simulink model "sampleModel1747_1_sub"  (R2023a)
settings: Solver=VariableStepAuto  StartTime=0.0  StopTime=10.0  RelTol=1e-3
libraries: hdlsllib x5, simulink x3
settings Model: Creator=user1  LastModifiedBy=user1

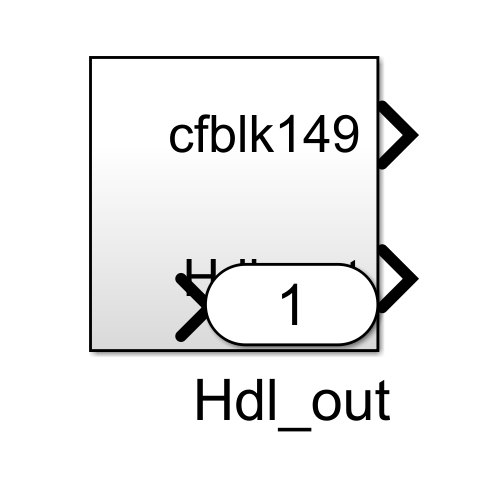
[thumbnail: Simulink's stored preview of the top-level diagram]
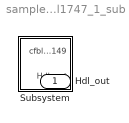
== system sampleModel1747_1_sub ==
  Subsystem : Subsystem
  Hdl_out : Outport  OutDataTypeStr=uint8

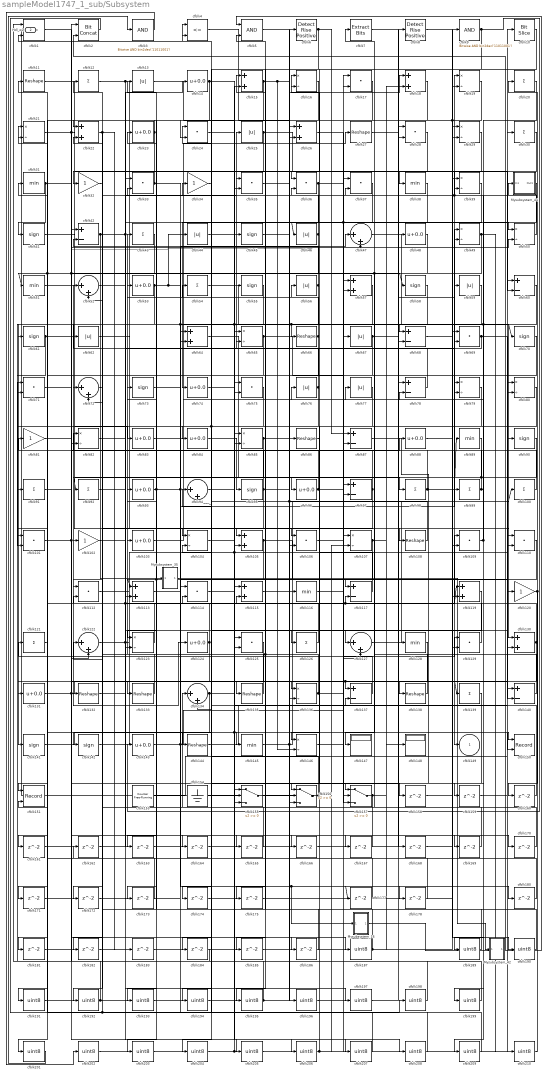
== system sampleModel1747_1_sub/Subsystem ==
  Mysubsystem_16 : Subsystem  TreatAsAtomicUnit=on  RTWFcnName=Mysubsystem_16
      settings: RTWFcnNameOpts=User specified  RTWFileNameOpts=Use function name
  Mysubsystem_35 : Subsystem  TreatAsAtomicUnit=on  RTWFcnName=Mysubsystem_35
      settings: RTWFcnNameOpts=User specified  RTWFileNameOpts=Use function name
  Mysubsystem_42 : Subsystem  TreatAsAtomicUnit=on  RTWFcnName=Mysubsystem_42
      settings: RTWFcnNameOpts=User specified  RTWFileNameOpts=Use function name
  Mysubsystem_44 : Subsystem  TreatAsAtomicUnit=on  RTWFcnName=Mysubsystem_44
      settings: RTWFcnNameOpts=User specified  RTWFileNameOpts=Use function name
  cfblk1 : RelationalOperator  Operator=<=  OutDataTypeStr=boolean  InputSameDT=off
  cfblk10 : hdlsllib/Logic and Bit Operations/Bit Slice  lidx=7  ridx=0
  cfblk{12,20,30,43,54,91..92,98..100,121,126,139} (13 alike) : Sum  Inputs=+  OutDataTypeStr=uint8
  cfblk{17,24,28,33,35..37,69,71,75,101,106,109..110,112,114,125,129} (18 alike) : DotProduct  OutDataTypeStr=uint8
  cfblk{32,34,81,102,120} (5 alike) : Gain  OutDataTypeStr=uint8
  cfblk{14,23,48,53,74,83..84,88,93,96,103,124,131,143} (14 alike) : Bias  Bias=0.0  SaturateOnIntegerOverflow=off
  cfblk{16,19,21,29,39,49..50,65,79..80,82,85,104,107,123,136,146} (17 alike) : Product  Inputs=*/  OutDataTypeStr=uint8  RndMeth=Zero  SaturateOnIntegerOverflow=on
  cfblk{15,18,22,26,57,64,105,113,115,119,130} (11 alike) : Sum  OutDataTypeStr=uint8
  cfblk{11,27,66,86,108,132..133,135,138,144} (10 alike) : Reshape
  cfblk{31,38,51,89,116,128,145} (7 alike) : MinMax  OutDataTypeStr=uint8
  cfblk{42,60,68,78,87,97,117,137,140} (9 alike) : Sum  Inputs=+-  OutDataTypeStr=uint8
  cfblk{47,52,72,94,122,127,134} (7 alike) : Sum  Inputs=|++  OutDataTypeStr=uint8
  cfblk{13,25,44,46,56,59,62,67,76..77} (10 alike) : Abs  OutDataTypeStr=uint8  SaturateOnIntegerOverflow=off
  cfblk{41,45,55,58,61,70,73,90,95,141..142} (11 alike) : Signum
  cfblk147 : Display
  cfblk148 : Display
  cfblk150 : Record  FileSettingsInternal="{\"entries\":[{\"content\":{\"excelSettings\":{\"content\":{},\"type\":\"Streamout.ExcelSettings\"}},\"type\":\"Streamout.FileSettingStorage\",\"uuid\":\"\"}],\"packageUris\":[\"http:\\/\\/schema.mathworks.com\\/mf0\\/streamout_blocks\\/R2020a\"],\"version\":\"1.0\"}"  Layout=[1 1]  SignalsInternal="{\"entries\":[{\"content\":{\"signals\":[{\"content\":{\"blockPath\":[],\"dimensions\":[1],\"domain\":\"\",\"lineColor\":\"#a2142f\",\"plots\":[1],\"port\":1,\"signalID\":39164,\"signalName\":\"cfblk36\"},\"type\":\"RecordBlkView.Signal\",\"uuid\":\"\"},{\"content\":{\"blockPath\":[],\"dimensions\":[1],\"domain\":\"\",\"lineColor\":\"#139fff\",\"plots\":[1],\"port\":2,\"signalID\":39167,\"signalName\":\"cfblk74\"},\"type\":\"RecordBlkView.Signal\",\"uuid\":\"\"}]},\"type\":\"RecordBlkView.InputSignals\",\"uuid\":\"\"}],\"packageUris\":[\"http:\\/\\/schema.mathworks.com\\/mf0\\/streamout_blocks\\/R2020a\"],\"version\":\"1.0\"}"  VisualizationBindings="{\"xyplotplugin\":{\"info\":[{\"series\":[{\"bindingParametersList\":[{\"parameter\":\"X-Axis\",\"signalID\":39164,\"signalName\":\"cfblk36\"},{\"parameter\":\"Y-Axis\",\"signalID\":39167,\"signalName\":\"cfblk74\"}],\"seriesID\":53810}],\"subplotID\":1}]}}"  CompatibilityTag=XY  st=-1
  cfblk151 : Record  FileSettingsInternal="{\"entries\":[{\"content\":{\"excelSettings\":{\"content\":{},\"type\":\"Streamout.ExcelSettings\"}},\"type\":\"Streamout.FileSettingStorage\",\"uuid\":\"\"}],\"packageUris\":[\"http:\\/\\/schema.mathworks.com\\/mf0\\/streamout_blocks\\/R2020a\"],\"version\":\"1.0\"}"  Layout=[1 1]  SignalsInternal="{\"entries\":[{\"content\":{\"signals\":[{\"content\":{\"blockPath\":[],\"dimensions\":[1],\"domain\":\"\",\"lineColor\":\"#a2142f\",\"plots\":[1],\"port\":1,\"signalID\":39156,\"signalName\":\"cfblk134\"},\"type\":\"RecordBlkView.Signal\",\"uuid\":\"\"},{\"content\":{\"blockPath\":[],\"dimensions\":[1],\"domain\":\"\",\"lineColor\":\"#139fff\",\"plots\":[1],\"port\":2,\"signalID\":39159,\"signalName\":\"cfblk209\"},\"type\":\"RecordBlkView.Signal\",\"uuid\":\"\"}]},\"type\":\"RecordBlkView.InputSignals\",\"uuid\":\"\"}],\"packageUris\":[\"http:\\/\\/schema.mathworks.com\\/mf0\\/streamout_blocks\\/R2020a\"],\"version\":\"1.0\"}"  VisualizationBindings="{\"xyplotplugin\":{\"info\":[{\"series\":[{\"bindingParametersList\":[{\"parameter\":\"X-Axis\",\"signalID\":39156,\"signalName\":\"cfblk134\"},{\"parameter\":\"Y-Axis\",\"signalID\":39159,\"signalName\":\"cfblk209\"}],\"seriesID\":64283}],\"subplotID\":1}]}}"  CompatibilityTag=XY  st=-1
  cfblk153 : hdlsllib/Sources/Counter Free-Running  NumBits=16  tsamp=-1
  cfblk154 : Ground
  cfblk155 : Switch  OutDataTypeStr=uint8  SaturateOnIntegerOverflow=off  InputSameDT=off
  cfblk156 : Switch  OutDataTypeStr=uint8  SaturateOnIntegerOverflow=off  InputSameDT=off
  cfblk157 : Switch  OutDataTypeStr=uint8  SaturateOnIntegerOverflow=off  InputSameDT=off
  cfblk{158..175,177..178,180..186} (27 alike) : Delay  SampleTime=1
  cfblk{187,189..199,201..210} (22 alike) : DataTypeConversion  OutDataTypeStr=uint8  SaturateOnIntegerOverflow=off  RndMeth=Floor
  cfblk2 : hdlsllib/Logic and Bit Operations/Bit Concat  numInputs=2
  cfblk3 : simulink/Logic and Bit Operations/Bitwise Operator  logicop=AND  UseBitMask=on  BitMask=bin2dec('11011001')  BitMaskRealWorld=Stored Integer
      settings: LibrarySourceBlock=|
      | hdlsllib/Logic and Bit
      | Operations/Bitwise
      | Operator
  cfblk4 : RelationalOperator  Operator=<=  OutDataTypeStr=boolean  InputSameDT=off
  cfblk5 : Logic  AllPortsSameDT=off  OutDataTypeStr=boolean
  cfblk6 : hdlsllib/Logic and Bit Operations/Detect Rise Positive  vinit=0  OutDataTypeStr=uint8
  cfblk7 : simulink/Logic and Bit Operations/Extract Bits  bitsToExtract=Upper half  numBits=8  bitIdxRange=[0 7]  outScalingMode=Preserve fixed-point scaling
      settings: LibrarySourceBlock=|
      | hdlsllib/Logic and Bit
      | Operations/Extract Bits
  cfblk8 : hdlsllib/Logic and Bit Operations/Detect Rise Positive  vinit=0  OutDataTypeStr=uint8
  cfblk9 : simulink/Logic and Bit Operations/Bitwise Operator  logicop=AND  UseBitMask=on  BitMask=bin2dec('11011001')  BitMaskRealWorld=Stored Integer
      settings: LibrarySourceBlock=|
      | hdlsllib/Logic and Bit
      | Operations/Bitwise
      | Operator
  cfblk149 : Outport  OutDataTypeStr=uint8  VectorParamsAs1DForOutWhenUnconnected=off
  Hdl_out : Outport  Port=2  OutDataTypeStr=uint8
  wires:
  cfblk83/1 -> cfblk27/1
  cfblk39/1 -> cfblk57/2, cfblk46/1
  cfblk12/1 -> cfblk50/1, cfblk98/1
  cfblk78/1 -> cfblk25/1
  cfblk87/1 -> cfblk157/1
  cfblk133/1 -> cfblk43/1
  cfblk157/1 -> cfblk148/1, cfblk134/1
  cfblk80/1 -> cfblk161/1, cfblk94/2
  cfblk17/1 -> cfblk203/1
  cfblk11/1 -> cfblk96/1
  cfblk84/1 -> cfblk95/1
  cfblk127/1 -> cfblk10/1
  cfblk31/1 -> cfblk41/1, cfblk138/1, cfblk58/1
  cfblk24/1 -> cfblk177/1, Mysubsystem_16/1(In1)
  cfblk62/1 -> cfblk108/1
  cfblk38/1 -> cfblk74/1
  cfblk79/1 -> cfblk156/1
  cfblk29/1 -> cfblk149/1
  cfblk61/1 -> cfblk101/2, cfblk124/1
  cfblk54/1 -> cfblk68/1
  cfblk156/1 -> Hdl_out/1, cfblk24/1
  cfblk46/1 -> cfblk22/2, cfblk181/1, cfblk51/1
  cfblk47/1 -> cfblk130/1
  cfblk75/1 -> cfblk141/1
  cfblk96/1 -> cfblk49/2, cfblk33/2
  cfblk25/1 -> cfblk113/2, cfblk38/1
  cfblk51/1 -> cfblk110/1
  cfblk4/1 -> cfblk86/1
  cfblk74/1 -> cfblk207/1, cfblk150/2
  cfblk146/1 -> cfblk157/2
  cfblk28/1 -> cfblk195/1
  cfblk145/1 -> cfblk77/1, cfblk49/1
  cfblk85/1 -> cfblk123/2, cfblk26/1
  cfblk130/1 -> cfblk172/1, cfblk15/1
  cfblk106/1 -> cfblk37/1
  cfblk103/1 -> cfblk6/1
  cfblk119/1 -> cfblk134/2
  cfblk49/1 -> cfblk210/1, cfblk87/2
  cfblk135/1 -> cfblk103/1
  cfblk89/1 -> cfblk106/1
  cfblk58/1 -> cfblk156/2
  cfblk123/1 -> cfblk11/1
  cfblk122/1 -> cfblk35/1, cfblk9/1
  cfblk55/1 -> cfblk91/1
  cfblk102/1 -> cfblk135/1
  cfblk137/1 -> cfblk121/1
  cfblk57/1 -> cfblk102/1
  cfblk94/1 -> cfblk55/1
  cfblk23/1 -> cfblk142/1, cfblk22/1
  cfblk120/1 -> cfblk160/1, Mysubsystem_44/1(In1)
  cfblk37/1 -> cfblk104/1
  cfblk142/1 -> cfblk80/1
  cfblk45/1 -> cfblk116/1
  cfblk14/1 -> cfblk178/1, cfblk24/2
  cfblk15/1 -> cfblk171/1, cfblk170/1, cfblk146/2
  cfblk109/1 -> cfblk199/1, cfblk79/2
  cfblk143/1 -> cfblk99/1, cfblk97/1
  cfblk144/1 -> cfblk80/2
  cfblk43/1 -> cfblk101/1
  cfblk105/1 -> cfblk173/1, cfblk140/1
  cfblk48/1 -> cfblk201/1, cfblk147/1
  cfblk19/1 -> cfblk119/2, cfblk123/1
  cfblk66/1 -> cfblk82/2, cfblk13/1
  cfblk69/1 -> cfblk65/2, cfblk120/1
  cfblk50/1 -> cfblk23/1, cfblk19/1
  cfblk126/1 -> cfblk73/1
  cfblk131/1 -> cfblk88/1, cfblk140/2
  cfblk141/1 -> cfblk145/1
  cfblk98/1 -> cfblk52/2, cfblk89/1
  cfblk138/1 -> cfblk82/1
  cfblk73/1 -> cfblk139/1, cfblk137/1
  cfblk112/1 -> cfblk15/2, cfblk29/1
  cfblk26/1 -> cfblk67/1
  cfblk124/1 -> cfblk112/2, cfblk133/1
  cfblk13/1 -> cfblk115/1
  cfblk93/1 -> cfblk53/1, cfblk47/1, cfblk105/2
  cfblk44/1 -> cfblk167/1, cfblk66/1, cfblk70/1
  cfblk32/1 -> cfblk132/1
  cfblk64/1 -> cfblk128/1
  cfblk18/1 -> cfblk61/1
  cfblk34/1 -> cfblk84/1
  cfblk108/1 -> cfblk54/1
  cfblk95/1 -> cfblk81/1, cfblk112/1, cfblk18/1
  cfblk9/1 -> cfblk36/1, cfblk143/1
  cfblk97/1 -> cfblk155/3, cfblk4/1
  cfblk20/1 -> cfblk209/1
  cfblk114/1 -> cfblk206/1
  cfblk41/1 -> cfblk83/1
  cfblk129/1 -> cfblk109/1
  cfblk125/1 -> cfblk192/1
  cfblk53/1 -> cfblk71/2, cfblk117/1, cfblk44/1
  cfblk70/1 -> cfblk131/1
  cfblk67/1 -> cfblk155/2, cfblk59/1
  cfblk154/1 -> cfblk137/2
  cfblk140/1 -> cfblk7/1
  cfblk1/1 -> cfblk122/2
  cfblk33/1 -> cfblk32/1, cfblk180/1, cfblk68/2
  cfblk121/1 -> cfblk21/1
  cfblk99/1 -> cfblk39/2, cfblk16/2, cfblk92/1
  cfblk82/1 -> cfblk130/2
  cfblk155/1 -> cfblk79/1, cfblk100/1
  cfblk65/1 -> cfblk127/2, cfblk144/1
  cfblk27/1 -> cfblk110/2
  cfblk42/1 -> cfblk14/1, cfblk127/1, Mysubsystem_35/1(In1)
  cfblk30/1 -> cfblk75/2
  cfblk153/1 -> cfblk90/1
  cfblk21/1 -> cfblk47/2, cfblk60/2
  cfblk72/1 -> cfblk12/1
  cfblk60/1 -> cfblk189/1, cfblk185/1
  cfblk117/1 -> cfblk56/1
  cfblk16/1 -> cfblk105/1
  cfblk22/1 -> cfblk183/1, cfblk182/1
  cfblk90/1 -> cfblk146/1
  cfblk76/1 -> cfblk52/1, cfblk163/1, cfblk113/1
  cfblk59/1 -> cfblk72/1
  cfblk77/1 -> cfblk157/3
  cfblk132/1 -> cfblk69/2, cfblk119/1, cfblk117/2
  cfblk136/1 -> cfblk129/1, cfblk115/2, cfblk72/2
  cfblk68/1 -> cfblk39/1
  cfblk101/1 -> cfblk158/1, cfblk50/2
  cfblk88/1 -> cfblk29/2
  cfblk36/1 -> cfblk194/1, cfblk150/1
  cfblk107/1 -> cfblk48/1, cfblk126/1
  cfblk56/1 -> cfblk174/1, cfblk42/2, cfblk16/1
  cfblk6/1 -> cfblk184/1, cfblk87/1
  cfblk134/1 -> cfblk151/1, cfblk76/1
  cfblk100/1 -> cfblk34/1
  cfblk5/1 -> cfblk187/1
  cfblk116/1 -> cfblk57/1
  cfblk86/1 -> cfblk136/1
  cfblk104/1 -> cfblk78/2
  cfblk158/1 -> cfblk129/2
  cfblk159/1 -> cfblk60/1
  cfblk160/1 -> cfblk1/2
  cfblk161/1 -> cfblk33/1
  cfblk162/1 -> cfblk75/1
  cfblk163/1 -> cfblk85/2
  cfblk52/1 -> cfblk164/1
  cfblk164/1 -> cfblk107/1
  cfblk113/1 -> cfblk165/1
  cfblk165/1 -> cfblk94/1
  cfblk71/1 -> cfblk166/1
  cfblk166/1 -> cfblk78/1
  cfblk167/1 -> cfblk122/1
  cfblk7/1 -> cfblk168/1
  cfblk168/1 -> cfblk109/2
  cfblk115/1 -> cfblk169/1
  cfblk169/1 -> cfblk65/1
  cfblk170/1 -> cfblk37/2
  cfblk171/1 -> cfblk64/1
  cfblk173/1 -> cfblk21/2
  cfblk174/1 -> cfblk106/2
  cfblk10/1 -> cfblk175/1
  cfblk175/1 -> cfblk69/1
  cfblk177/1 -> cfblk104/2
  cfblk178/1 -> cfblk42/1
  cfblk180/1 -> cfblk4/2
  cfblk181/1 -> cfblk26/2
  cfblk182/1 -> cfblk97/2
  cfblk183/1 -> cfblk19/2
  cfblk184/1 -> cfblk1/1
  cfblk185/1 -> cfblk136/2
  cfblk81/1 -> cfblk186/1
  cfblk186/1 -> cfblk155/1
  cfblk187/1 -> cfblk18/2, cfblk62/1
  cfblk189/1 -> cfblk5/2
  cfblk8/1 -> cfblk190/1
  cfblk190/1 -> cfblk93/1
  cfblk128/1 -> cfblk191/1
  cfblk191/1 -> cfblk8/1
  cfblk192/1 -> cfblk71/1, cfblk64/2
  cfblk110/1 -> cfblk193/1
  cfblk193/1 -> cfblk125/1
  cfblk194/1 -> cfblk125/2
  cfblk195/1 -> cfblk31/1, cfblk156/3
  cfblk35/1 -> cfblk196/1
  cfblk196/1 -> cfblk28/1
  cfblk92/1 -> cfblk197/1
  cfblk197/1 -> cfblk28/2
  cfblk2/1 -> cfblk198/1
  cfblk198/1 -> cfblk85/1
  cfblk199/1 -> cfblk2/1
  cfblk201/1 -> cfblk3/1
  cfblk3/1 -> cfblk202/1
  cfblk202/1 -> cfblk45/1
  cfblk203/1 -> cfblk30/1, cfblk35/2
  cfblk139/1 -> cfblk204/1
  cfblk204/1 -> cfblk17/1
  cfblk91/1 -> cfblk205/1
  cfblk205/1 -> cfblk17/2
  cfblk206/1 -> cfblk107/2, cfblk36/2
  cfblk207/1 -> cfblk114/1
  cfblk172/1 -> cfblk208/1
  cfblk208/1 -> cfblk114/2
  cfblk209/1 -> cfblk151/2, cfblk162/1
  cfblk210/1 -> cfblk20/1
  Mysubsystem_16/1(Out1) -> cfblk5/1
  Mysubsystem_35/1(Out1) -> Mysubsystem_42/1(In1)
  Mysubsystem_42/1(Out1) -> cfblk2/2
  Mysubsystem_44/1(Out1) -> cfblk159/1

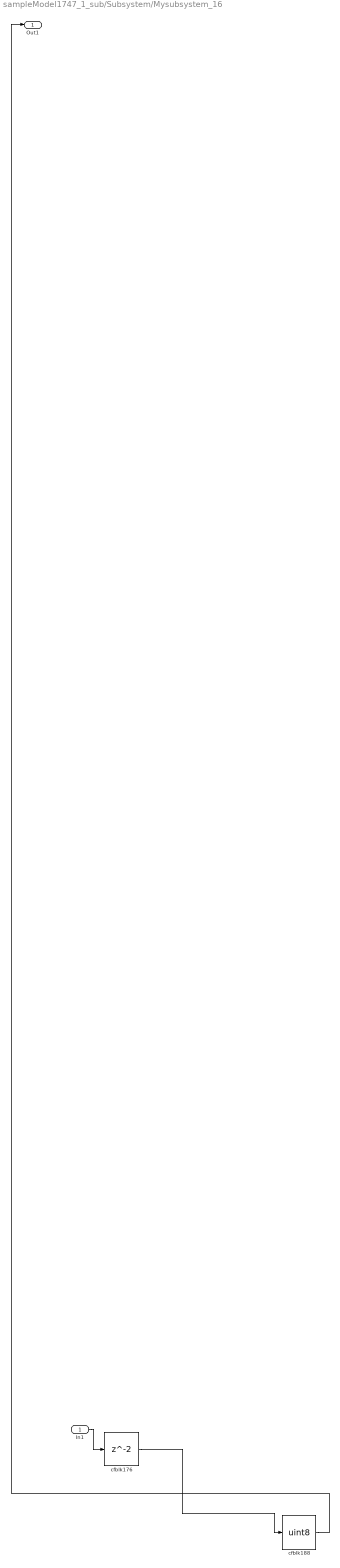
== system sampleModel1747_1_sub/Subsystem/Mysubsystem_16 ==
  In1 : Inport
  cfblk176 : Delay  SampleTime=1
  cfblk188 : DataTypeConversion  OutDataTypeStr=uint8  SaturateOnIntegerOverflow=off  RndMeth=Floor
  Out1 : Outport
  wires:
  cfblk188/1 -> Out1/1
  In1/1 -> cfblk176/1
  cfblk176/1 -> cfblk188/1

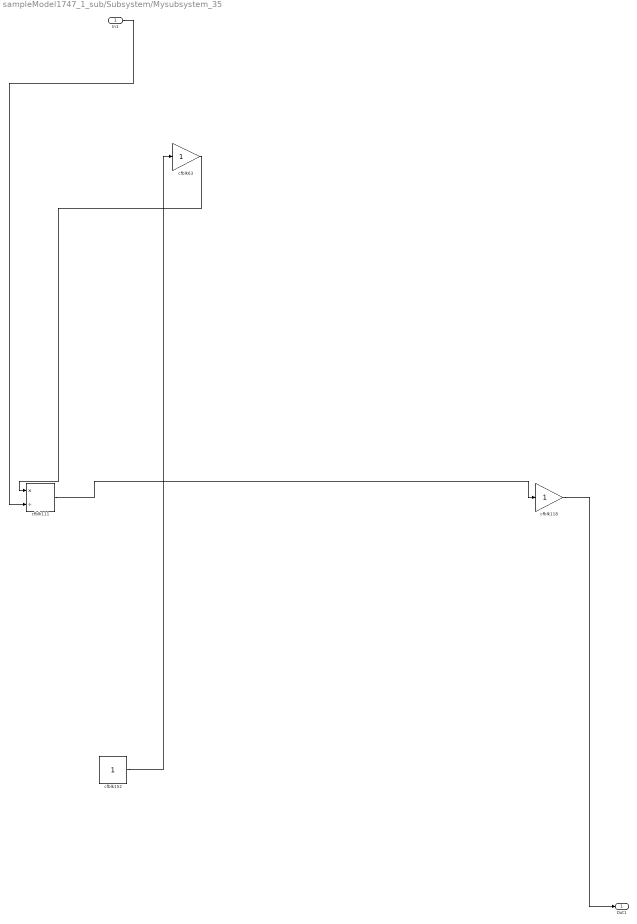
== system sampleModel1747_1_sub/Subsystem/Mysubsystem_35 ==
  In1 : Inport
  cfblk111 : Product  Inputs=*/  RndMeth=Zero  SaturateOnIntegerOverflow=on
  cfblk118 : Gain
  cfblk152 : Constant  SampleTime=-1
  cfblk63 : Gain
  Out1 : Outport
  wires:
  cfblk118/1 -> Out1/1
  cfblk63/1 -> cfblk111/1
  In1/1 -> cfblk111/2
  cfblk152/1 -> cfblk63/1
  cfblk111/1 -> cfblk118/1

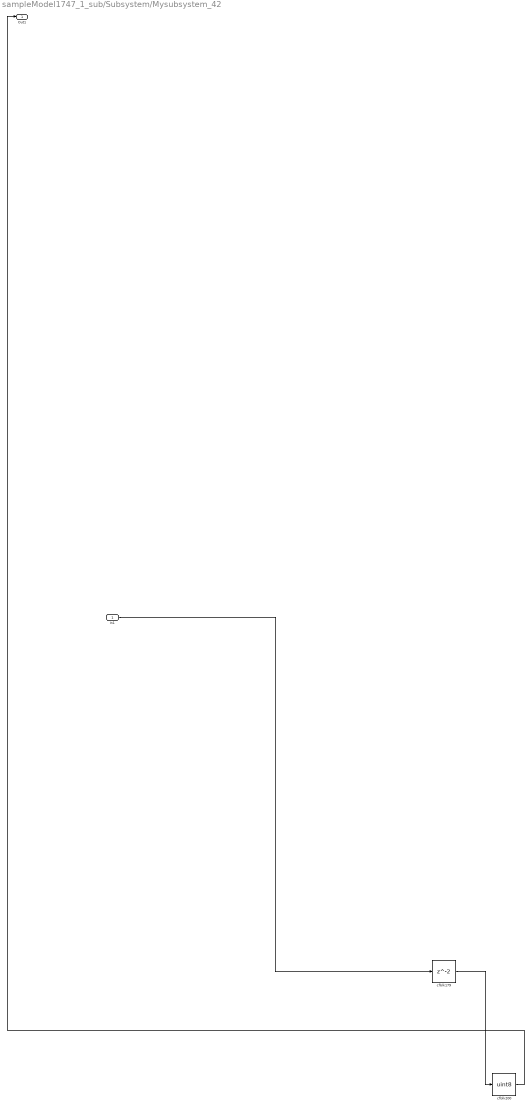
== system sampleModel1747_1_sub/Subsystem/Mysubsystem_42 ==
  In1 : Inport
  cfblk179 : Delay  SampleTime=1
  cfblk200 : DataTypeConversion  OutDataTypeStr=uint8  SaturateOnIntegerOverflow=off  RndMeth=Floor
  Out1 : Outport
  wires:
  cfblk200/1 -> Out1/1
  In1/1 -> cfblk179/1
  cfblk179/1 -> cfblk200/1

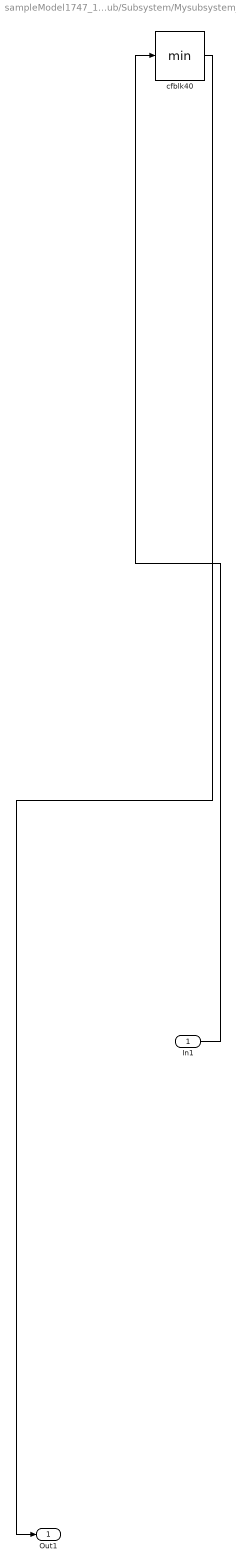
== system sampleModel1747_1_sub/Subsystem/Mysubsystem_44 ==
  In1 : Inport
  cfblk40 : MinMax
  Out1 : Outport
  wires:
  cfblk40/1 -> Out1/1
  In1/1 -> cfblk40/1
